simulink model "model_verification"  (Simulink 10.2)
settings: Solver=ode1  StartTime=0.0  StopTime=35  FixedStep=0.002  RelTol=1e-3  EnableMultiTasking=on
PreLoadFcn:
  | quanser_aero_lqr
undefined symbols (not defined in the file or in its folder): HIL, qc_get_step_size
libraries: quarc_library x4
settings Model: Creator=MLevis  LastModifiedBy=ffsandva  SimulationMode=external  ExtModeTrigDuration=20000
settings SolverCC: PositivePriorityOrder=on
settings DataIOCC: LimitDataPoints=on  SignalLoggingSaveFormat=Dataset
settings DebuggingCC: UnderspecifiedInitializationDetection=Simplified  MergeDetectMultiDrivingBlocksExec=error  SolverPrmCheckMsg=warning  FcnCallInpInsideContextMsg=error
settings RTWCC: Description=QUARC Win64 Target  SystemTargetFile=quarc_win64.tlc  TemplateMakefile=quarc_default_tmf
settings STFCustomTargetCC: TargetPreCompLibLocation=C:\PROGRA~3\QUARC\lib\2020b\win64\release  ConcurrentExecutionCompliant=on  SystemTargetFile=quarc_win64.tlc
settings GRTTargetCC: TargetPreCompLibLocation=C:\PROGRA~3\QUARC\lib\2020b\win64\release  ParMdlRefBuildCompliant=off  CompOptLevelCompliant=off  MatFileLogging=off  CPPClassGenCompliant=off  UseToolchainInfoCompliant=off  ExtMode=on  ExtModeMexFile=quarc_comm
settings ConfigComp: CovSFcnEnable=off

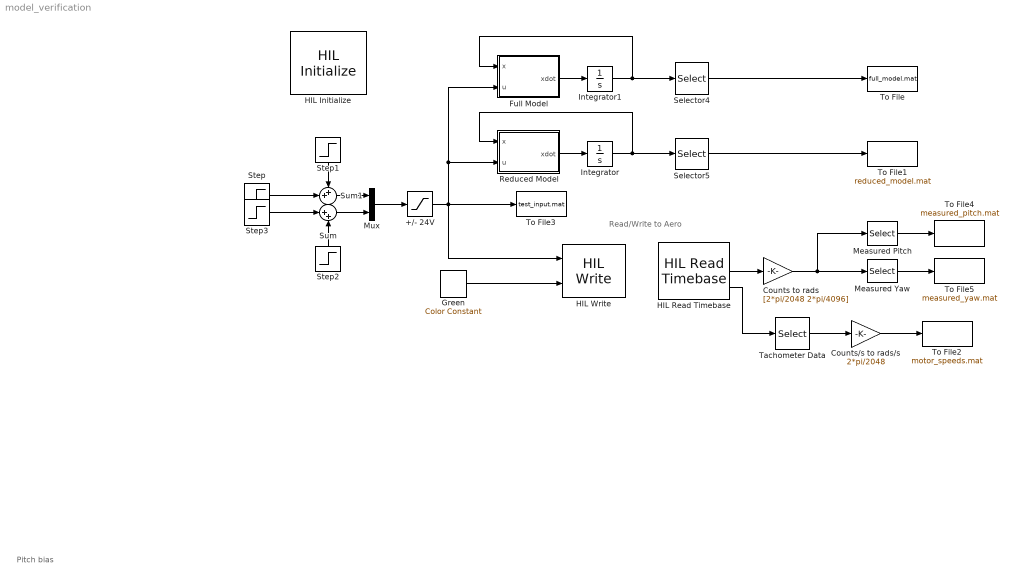
== system model_verification ==
  note: Read/Write to Aero
  note: Pitch bias
  +/- 24V : Saturate  UpperLimit=24  LowerLimit=-24
  Counts to rads : Gain  Gain=[2*pi/2048 2*pi/4096]
  Counts/s to rads/s : Gain  Gain=2*pi/2048
  Full Model : MATLAB Function  TreatAsAtomicUnit=on
  Green : quarc_library/Sources/Signals/Color Constant  color=[0 1 0]
      settings: SourceProductName=QUARC Targets
  HIL Initialize : quarc_library/Data Acquisition/Generic/Configuration/HIL Initialize  Priority=-99  object_name=HIL-1  board_type=quanser_aero_usb  board_number=0  board_options=""  exclusive=off  active=off  hardware_clocks=[0]  clock_modes=[]  initial_clock_frequencies=[]  set_clock_params_at_start=off  set_clock_params_at_switch_in=off  set_clock_frequencies_at_start=off  set_clock_frequencies_at_switch_in=off  analog_input_channels=[0:1]  analog_input_configurations=[]  analog_input_maximums=3  analog_input_minimums=-3  set_analog_input_params_at_start=off  set_analog_input_params_at_switch_in=off  analog_output_channels=[0:1]  analog_output_maximums=24  analog_output_minimums=-24  initial_analog_outputs=[0]  final_analog_outputs=[0]  watchdog_analog_outputs=[0]  set_analog_output_params_at_start=off  set_analog_output_params_at_switch_in=off  set_analog_outputs_at_start=on  set_analog_outputs_at_switch_in=off  set_analog_outputs_at_terminate=on  set_analog_outputs_at_switch_out=off  set_analog_outputs_on_watchdog=on  digital_input_channels=[]  digital_output_channels=[0:1]  digital_output_configuration=[]  initial_digital_outputs=[1]  final_digital_outputs=[0]  watchdog_digital_outputs=[0]  set_digital_output_params_at_start=off  set_digital_output_params_at_switch_in=off  set_digital_outputs_at_start=on  set_digital_outputs_at_switch_in=off  set_digital_outputs_at_terminate=on  set_digital_outputs_at_switch_out=off  set_digital_outputs_on_watchdog=on  encoder_channels=[0:3]  quadrature=[4]  encoder_filter_frequency=[]  initial_encoder_counts=[0]  set_encoder_params_at_start=off  set_encoder_params_at_switch_in=off  set_encoder_counts_at_start=on  set_encoder_counts_at_switch_in=off  pwm_channels=[]  pwm_modes=[]  pwm_frequency=[]  pwm_configuration=[]  pwm_alignment=[]  pwm_polarity=[]  pwm_leading_deadband=[]  pwm_trailing_deadband=[]  initial_pwm_outputs=[]  final_pwm_outputs=[]  watchdog_pwm_outputs=[]  set_pwm_params_at_start=off  set_pwm_params_at_switch_in=off  set_pwm_outputs_at_start=off  set_pwm_outputs_at_switch_in=off  set_pwm_outputs_at_terminate=off  set_pwm_outputs_at_switch_out=off  set_pwm_outputs_on_watchdog=off  other_output_channels=[11000:11002]  initial_other_outputs=[0 1 0]  final_other_outputs=[1 0 0]  watchdog_other_outputs=[0 0 1]  set_other_outputs_at_start=on  set_other_outputs_at_switch_in=off  set_other_outputs_at_terminate=on  set_other_outputs_at_switch_out=off  set_other_outputs_on_watchdog=on
  HIL Read Timebase : quarc_library/Data Acquisition/Generic/Timebases/HIL Read Timebase  object_name=HIL-1  clock=0  analog_channels=[0:1]  encoder_channels=[2:3]  digital_channels=[]  other_channels=[4000 4002 14000 14001]  active=on  vector_output=on  data_type_mode=Inherit via back propagation  encoder_data_type=double  digital_data_type=boolean  overflow_mode=Error on overflow  samples_in_buffer=max(ceil(1/qc_get_step_size), 1)
  HIL Write : quarc_library/Data Acquisition/Generic/Immediate I//O/HIL Write  object_name=HIL-1  analog_channels=[0:1]  pwm_channels=[]  digital_channels=[]  other_channels=[11000:11002]  sample_time=-1  active=off  vector_input=on
  Integrator : Integrator
  Integrator1 : Integrator
  Measured Pitch : Selector  InputPortWidth=2  IndexOptions=Index vector (dialog)  Indices=[1]  OutputSizes=1
  Measured Yaw : Selector  InputPortWidth=2  IndexOptions=Index vector (dialog)  Indices=[2]  OutputSizes=1
  Mux : Mux  Inputs=2
  Reduced Model : MATLAB Function  TreatAsAtomicUnit=on
  Selector4 : Selector  InputPortWidth=4  IndexOptions=Index vector (dialog)  Indices=[1 2]  OutputSizes=1
  Selector5 : Selector  InputPortWidth=4  IndexOptions=Index vector (dialog)  Indices=[1 2]  OutputSizes=1
  Step : Step  Time=5  After=10  SampleTime=0
  Step1 : Step  Time=15  After=-10  SampleTime=0
  Step2 : Step  Time=25  After=-10  SampleTime=0
  Step3 : Step  Time=15  After=10  SampleTime=0
  Sum : Sum  Inputs=|++
  Sum1 : Sum  Inputs=++|
  Tachometer Data : Selector  InputPortWidth=4  IndexOptions=Index vector (dialog)  Indices=[3 4]  OutputSizes=1
  To File : ToFile  Filename=full_model.mat  MatrixName=full_model
  To File1 : ToFile  Filename=reduced_model.mat  MatrixName=reduced_model
  To File2 : ToFile  Filename=motor_speeds.mat  MatrixName=motor_speeds
  To File3 : ToFile  Filename=test_input.mat  MatrixName=test_input
  To File4 : ToFile  Filename=measured_pitch.mat  MatrixName=measured_pitch
  To File5 : ToFile  Filename=measured_yaw.mat  MatrixName=measured_yaw
  wires:
  Mux/1 -> +/- 24V/1
  HIL Read Timebase/2 -> Counts to rads/1
  +/- 24V/1 -> Full Model/2(u), Reduced Model/2(u), To File3/1, HIL Write/1
  Green/1 -> HIL Write/2
  Counts to rads/1 -> Measured Pitch/1, Measured Yaw/1
  HIL Read Timebase/3 -> Tachometer Data/1
  Counts/s to rads/s/1 -> To File2/1
  Tachometer Data/1 -> Counts/s to rads/s/1
  Sum/1 -> Mux/2
  Sum1/1 -> Mux/1
  Step/1 -> Sum1/2
  Step1/1 -> Sum1/1
  Step3/1 -> Sum/1
  Step2/1 -> Sum/2
  Reduced Model/1(xdot) -> Integrator/1
  Integrator1/1 -> Full Model/1(x), Selector4/1
  Full Model/1(xdot) -> Integrator1/1
  Selector4/1 -> To File/1
  Selector5/1 -> To File1/1
  Integrator/1 -> Reduced Model/1(x), Selector5/1
  Measured Pitch/1 -> To File4/1
  Measured Yaw/1 -> To File5/1

== matlab function Full Model ==
  data: x input double; u input double; xdot output double
function xdot = FullModel(x, u)
    utilde = [
        u(1)^2;
        u(2)^2;
    ];
    theta = x(1);
    psi = x(2);
    thetadot = x(3);
    psidot = x(4);
    
    % parameters
    g = 9.81;
    dt = 0.158;
    me = 0.2;
    dx = 0.016;
    
    ry = 0.02;
    my = 0.526;
    
    mpa = 0.146;
    lt = 0.165;
    mmt = 0.089;
    mtt = 0.089;
    mtc = 0.280;
    mrod = mmt + mtt + mtc;
    
    Ibxx = 2*me*dx^2;
    Ibxy = me*dt*dx;
    Ibyy = 2*mpa*dt^2 + 2*me*dt^2 + me*dx^2 + 1/12*mrod*lt^2;
    Ifyzz = 1/2*my*ry^2;
    
    Komega = 17.38;
    
    M = [
        Ibyy, -Ibxy * sin(theta);
        -Ibxy * sin(theta), Ifyzz + Ibxy * sin(2*theta) + 0.5*(Ibxx + Ibyy + (Ibyy - Ibxx)*cos(2*theta));
    ];
    C = [
        0, Ibxy*psidot*(1-2*cos(theta)^2) + (Ibyy-Ibxx)*psidot*cos(theta)*sin(theta);
        -Ibxy*thetadot*cos(theta), 2*Ibxy*thetadot*cos(2*theta) + 2*(Ibxy-Ibyy)*thetadot*cos(theta)*sin(theta);
    ];
    gvec = [
        dx * g * me * sin(theta);
        0;
    ];
    
    Kmtheta = 1.26e-6;
    Kttheta = 1.08e-6;
    Ktpsi = Kmtheta;
    Kmpsi = Kttheta;

    B = Komega^2 * [
        dt * Kmtheta, dt * Kttheta;
        -dt * Kmpsi * cos(theta), dt * Ktpsi * cos(theta);
    ];

    dtheta = 0.0031;
    dpsi = 0.0075;
    D = [
        dtheta, 0;
        0, dpsi;
    ];

    q = [
        theta;
        psi;
    ];
    qdot = [
        thetadot;
        psidot;
    ];

    xdot = [
        qdot;
        M \ (B*utilde - C*qdot - D*qdot - gvec);
    ];
end

== matlab function Reduced Model ==
  data: x input double; u input double; xdot output double
function xdot = ReducedModel(x, u)
    utilde = [
        u(1)^2;
        u(2)^2;
    ];
    theta = x(1);
    psi = x(2);
    thetadot = x(3);
    psidot = x(4);
    
    % parameters
    g = 9.81;
    dt = 0.158;
    me = 0.2;
    dx = 0.016;
    
    ry = 0.02;
    my = 0.526;
    
    mpa = 0.146;
    lt = 0.165;
    mmt = 0.089;
    mtt = 0.089;
    mtc = 0.280;
    mrod = mmt + mtt + mtc;
    
    Ibyy = 2*mpa*dt^2 + 2*me*dt^2 + me*dx^2 + 1/12*mrod*lt^2;
    Ifyzz = 1/2*my*ry^2;
    
    Komega = 17.38;

    M = [
        Ibyy, 0;
        0, Ifyzz + Ibyy * cos(theta)^2;
    ];
    C = [
        0, Ibyy * psidot * cos(theta)*sin(theta);
        0, -2*Ibyy * thetadot * cos(theta)*sin(theta);
    ];
    gvec = [
        dx * g * me * sin(theta);
        0;
    ];
    
    Kmtheta = 1.26e-6;
    Kttheta = 1.08e-6;
    Ktpsi = Kmtheta;
    Kmpsi = Kttheta;

    B = Komega^2 * [
        dt * Kmtheta, dt * Kttheta;
        -dt * Kmpsi * cos(theta), dt * Ktpsi * cos(theta);
    ];

    dtheta = 0.0031;
    dpsi = 0.0075;
    D = [
        dtheta, 0;
        0, dpsi;
    ];

    q = [
        theta;
        psi;
    ];
    qdot = [
        thetadot;
        psidot;
    ];

    xdot = [
        qdot;
        M \ (B*utilde - C*qdot - D*qdot - gvec);
    ];
end
